simulink model "Control_Block_2"  (R2022a)
settings: Solver=FixedStepAuto  StartTime=0.0  StopTime=end_time  FixedStep=dt  RelTol=1e-3
values from neighbouring files (symbols this model uses):
  Area = pi() * r0^2    [Main_PD_Control.m]    (also in Test_code.m; main.m = 1.25663706144e-05; main2.m = 1.25663706144e-05)
  Cd = 0.42    [Main_PD_Control.m]    (also in Test_code.m; main.m = 1.05; main2.m = 1.05)
  dt = 0.01    [Main_PD_Control.m]    (also in Test_code.m; load_parameter.m; main.m; main2.m = 0.001)
  K_d = 10    [Main_PD_Control.m]    (also in Test_code.m = 0; main.m; main2.m)
  K_p = 100    [Main_PD_Control.m]    (also in Test_code.m; main.m = 500; main2.m)
  rho_blood = 1025    [main.m]    (also in main2.m)
settings Model: Creator=zhong  LastModifiedBy=normanzmz
settings DebuggingCC: UnconnectedInputMsg=warning  UnconnectedOutputMsg=warning  UnconnectedLineMsg=warning
settings RTWCC: DLArmComputeVersion=19.05

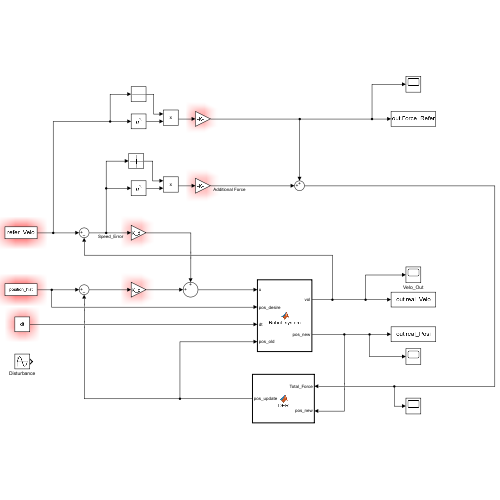
[thumbnail: Simulink's stored preview of the top-level diagram]
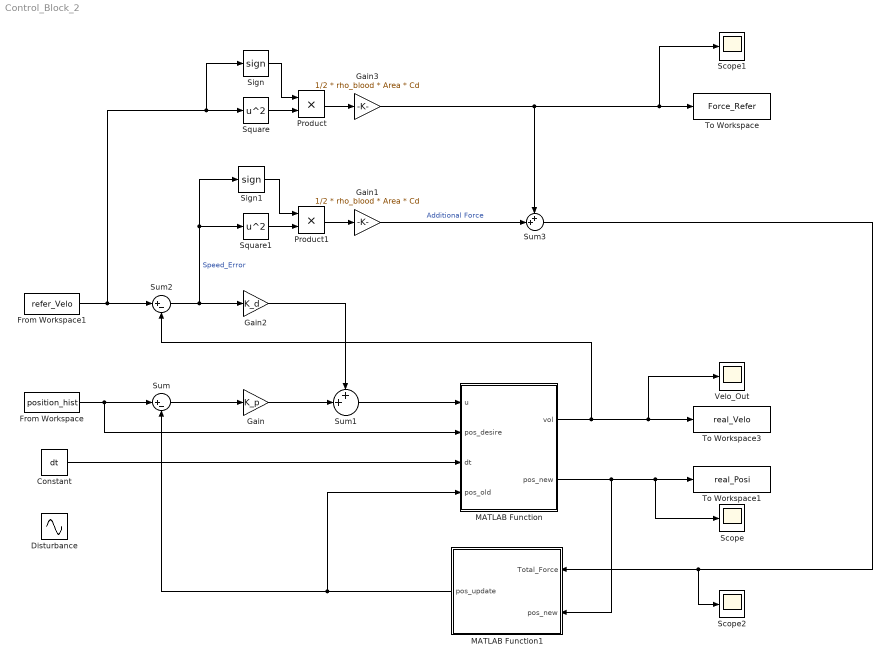
== system Control_Block_2 ==
  Constant : Constant  Value=dt
  Disturbance : Sin  Amplitude=2  Frequency=10  SampleTime=0
  From Workspace : FromWorkspace  VariableName=position_hist
  From Workspace1 : FromWorkspace  VariableName=refer_Velo
  Gain : Gain  Gain=K_p
  Gain1 : Gain  Gain=1/2 * rho_blood * Area * Cd
  Gain2 : Gain  Gain=K_d
  Gain3 : Gain  Gain=1/2 * rho_blood * Area * Cd
  MATLAB Function : MATLAB Function  TreatAsAtomicUnit=on
  MATLAB Function1 : MATLAB Function  TreatAsAtomicUnit=on
  Product : Product
  Product1 : Product
  Scope : Scope
  Scope1 : Scope
  Scope2 : Scope
  Sign : Signum
  Sign1 : Signum
  Square : Math  Operator=square
  Square1 : Math  Operator=square
  Sum : Sum  Inputs=|+-
  Sum1 : Sum  Inputs=++|
  Sum2 : Sum  Inputs=|+-
  Sum3 : Sum  Inputs=++|
  To Workspace : ToWorkspace  VariableName=Force_Refer  SaveFormat=Structure With Time  SampleTime=-1
  To Workspace1 : ToWorkspace  VariableName=real_Posi  SaveFormat=Timeseries  SampleTime=-1
  To Workspace3 : ToWorkspace  VariableName=real_Velo  SaveFormat=Timeseries  SampleTime=-1
  Velo_Out : Scope
  wires:
  From Workspace/1 -> MATLAB Function/2(pos_desire), Sum/1
  Sum/1 -> Gain/1
  Gain/1 -> Sum1/2
  Sum2/1 -> Sign1/1, Square1/1, Gain2/1  "Speed_Error"
  Gain2/1 -> Sum1/1
  Sum1/1 -> MATLAB Function/1(u)
  From Workspace1/1 -> Sum2/1, Sign/1, Square/1
  Sum3/1 -> MATLAB Function1/1(Total_Force), Scope2/1
  Constant/1 -> MATLAB Function/3(dt)
  MATLAB Function/2(pos_new) -> MATLAB Function1/2(pos_new), Scope/1, To Workspace1/1
  MATLAB Function/1(vol) -> Sum2/2, Velo_Out/1, To Workspace3/1
  Gain3/1 -> Sum3/1, Scope1/1, To Workspace/1
  Gain1/1 -> Sum3/2  "Additional Force"
  Square/1 -> Product/2
  Sign/1 -> Product/1
  Product/1 -> Gain3/1
  Sign1/1 -> Product1/1
  Square1/1 -> Product1/2
  Product1/1 -> Gain1/1
  MATLAB Function1/1(pos_update) -> MATLAB Function/4(pos_old), Sum/2

== matlab function Control_Block_2/MATLAB Function1 ==
  data: Total_Force input; pos_update output; pos_new input
function pos_update = DER(Total_Force,pos_new)
%% Time setup
total_Time = 5;
dt = 0.01;
N_step = total_Time / dt;

%% Beam parameters 
N = 50; % Number of nodes 
l = 0.5; % beam length
R = 0.002; % beam outer radius 
r = 0.001; % beam inner radius
rho_beam = 980; % PDMS density
E = 1.47e6; % Youngs Modulus

dl = l / (N - 1); % length of each segment 
A = pi*(R^2-r^2); % Beam cross-section 

m = A*l*rho_beam/(N-1); % mass of each node  
I = pi/4*(R^4 - r^4); % Moment of inerita 

EA = E*A; % Stretching stiffness 
EI = E*I; % Bending stiffness 

% Beam Mass Matrix 
M = zeros(2*N,2*N);
for i = 1 : 2*N
    M(i,i) = m;
end 
%% Beam initial configuration 
% Initial position 
nodes_I = zeros(N,2);
for i = 1:N 
    nodes_I(i,1) = (1-i) * dl + init_pos;
    nodes_I(i,2) = init_pos;
end 

% Initial DOF vector
q0 = zeros(2*N,1);
for i = 1:N
    q0 (2*i-1) = nodes_I(i,1); % x coordinate 
    q0 (2*i) = nodes_I(i,2); % y coordinate
end

% Initial position and velo 
q = q0;
u = (q - q0) / dt;

% tolerance 
tol = EI / l^2 * 1e-3; 
Ex_force = zeros(2*N,1);
    
    err = 10 * tol;
    % Newton Raphson
    while err > tol

    % Inertia 
    f = M/dt * ((q - q0) / dt - u);
    J = M/ dt^2;

    % Elastic forces 
    % Linear Spring 1 between node 1 and 2
    for k = 1: N-1
        xk = q(2*k-1);
        yk = q(2*k);
        xkp1 = q(2*k+1);
        ykp1 = q(2*k+2); 
        dF = gradEs(xk, yk, xkp1, ykp1, dl, EA);
        dJ = hessEs(xk, yk, xkp1, ykp1, dl, EA);
        f(2*k-1:2*k+2) = f(2*k-1:2*k+2) + dF;
        J(2*k-1:2*k+2, 2*k-1:2*k+2) = ...
        J(2*k-1:2*k+2, 2*k-1:2*k+2) + dJ;
    end

    % Bending spring 
    for k = 2:N-1
        xkm1 = q(2*k-3);
        ykm1 = q(2*k-2);
        xk = q(2*k-1);
        yk = q(2*k);
        xkp1 = q(2*k+1);
        ykp1 = q(2*k+2);
        curvature0 = 0;
        dF = gradEb(xkm1, ykm1, xk, yk, xkp1, ykp1, curvature0, dl, EI);
        dJ = hessEb(xkm1, ykm1, xk, yk, xkp1, ykp1, curvature0, dl, EI);
        f(2*k-3:2*k+2) = f(2*k-3:2*k+2) + dF;
        J(2*k-3:2*k+2, 2*k-3:2*k+2) = ...
            J(2*k-3:2*k+2, 2*k-3:2*k+2) + dJ;
    end
    
    % External force 
    Ex_force(1) = Total_Force(1);
    Ex_force(2) = Total_Force(2);

    % Weight 
    f = f + Ex_force;

    % Update 
    q(1:(2*N)) = q(1:(2*N)) - J(1:(2*N),1:(2*N)) \ f(1:(2*N));
    err = sum(abs(f(1:(2*N))));
    end

    % Update
    u = (q - q0) / dt;
    q0 = q;
    
    % plot of sphere position
    figure(1);
    plot(result(:,1),result(:,2), 'y');
    hold on
    plot(lines(:,1),lines(:,2), 'b');
    hold on
    plot(q(1:2:end),q(2:2:end),'ro-');
    plot(real_Posi(i,1), real_Posi(i,2),'ro');
%   axis equal
    axis([-0.5,1.1,-0.1,1.1])
    hold off
    drawnow
end 

end

== matlab function Control_Block_2/MATLAB Function ==
  data: vol output; u input; pos_desire input; dt input; pos_old input; pos_new output
function [vol,pos_new] = Robot_system(u,pos_desire,dt,pos_old)

pos_new = pos_desire + u;

vol = (pos_new - pos_old)/dt;
